simulink model "HW0X03Sim"  (R2021b)
settings: Solver=VariableStepAuto  StartTime=0.0  StopTime=1  RelTol=1e-3
undefined symbols (not defined in the file): A, B, K, state_var, Tx
settings Model: Creator=cclep  LastModifiedBy=cclep
settings SolverCC: AlgebraicLoopSolver=TrustRegion
settings DebuggingCC: SFMachineParentedDataDiag=warning

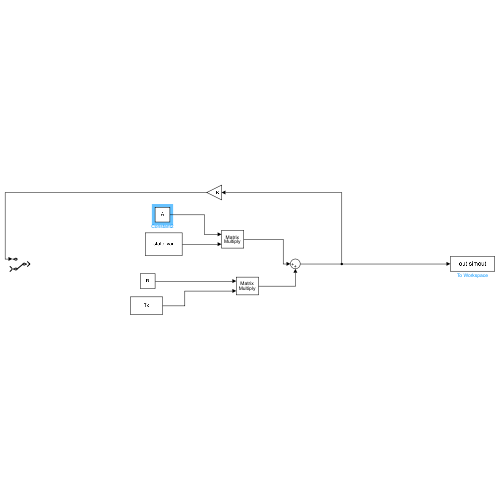
[thumbnail: Simulink's stored preview of the top-level diagram]
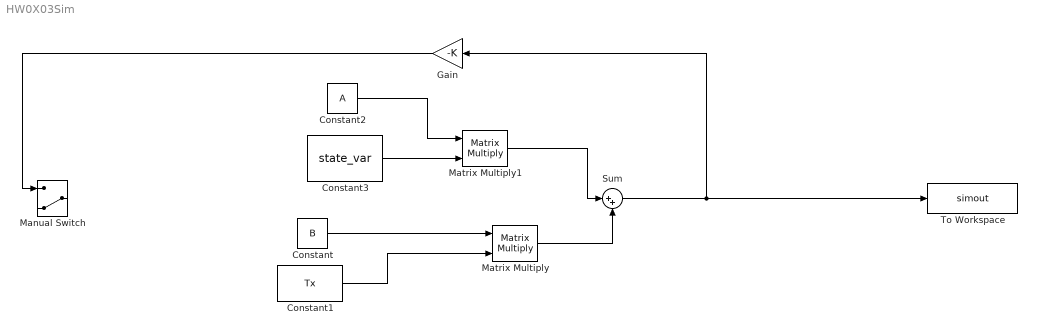
== system HW0X03Sim ==
  Constant : Constant  Value=B
  Constant1 : Constant  Value=Tx
  Constant2 : Constant  Value=A
  Constant3 : Constant  Value=state_var  VectorParams1D=off
  Gain : Gain  Gain=-K
  Manual Switch : ManualSwitch  CurrentSetting=0
  Matrix Multiply : Product  Multiplication=Matrix(*)
  Matrix Multiply1 : Product  Multiplication=Matrix(*)
  Sum : Sum  Inputs=|++
  To Workspace : ToWorkspace  VariableName=simout  SampleTime=-1
  wires:
  Constant/1 -> Matrix Multiply/1
  Constant3/1 -> Matrix Multiply1/2
  Constant2/1 -> Matrix Multiply1/1
  Matrix Multiply1/1 -> Sum/1
  Matrix Multiply/1 -> Sum/2
  Sum/1 -> Gain/1, To Workspace/1
  Constant1/1 -> Matrix Multiply/2
  Gain/1 -> Manual Switch/1
